simulink model "MZ0x2DH1921_EV_Personalise_design_witthmotor"  (R2023b)
settings: Solver=VariableStepAuto  StartTime=0.0  StopTime=100  RelTol=1e-3
libraries: spsDCVoltageSourceLib x3, spsDCMachineLib x2, spsControlledVoltageSourceLib x1, sps_lib x1
settings Model: Creator=HP5CD  LastModifiedBy=HP5CD

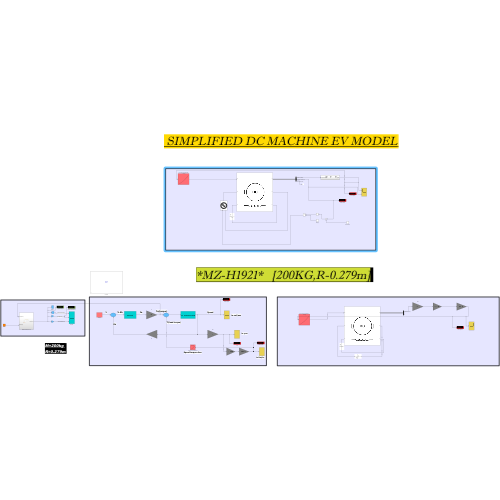
[thumbnail: Simulink's stored preview of the top-level diagram]
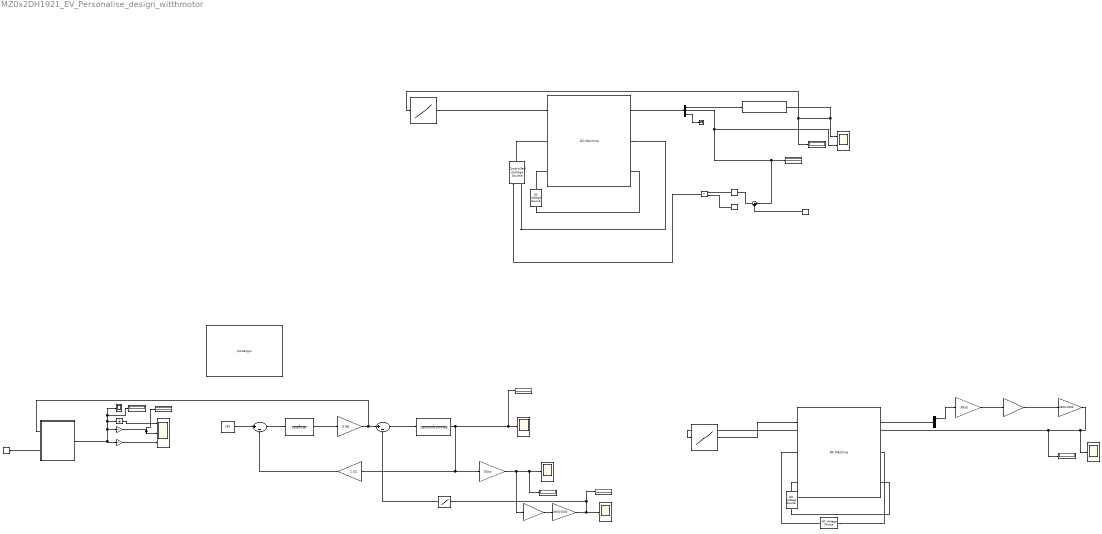
== system MZ0x2DH1921_EV_Personalise_design_witthmotor ==
  note: SIMPLIFIED DC MACHINE EV MODEL
  note: Speed torque-char
  note: in Km/hr
  note: in rpm
  note: in rad/sec
  note: Speed
  note: Tl(load torque)
  note: Te(torque)
  note: Ia
  note: V-Eb
  note: Eb
  note: V
  note: *MZ-H1921* [200KG,R-0.279m]
  note: Distance Covered(m)
  note: M=200kg
      | R=0.279m
  note: Speed(Km/hr)
  "                " : Gain  Gain=3600/1000
  "                Wheel RPM(no gear)" : Gain  Gain=60/(2.3*2*0.279)
  200KG Vehicle ,R=0.279 : Subsystem
  Bus Selector : BusSelector  OutputSignals=Speed wm (rad/s),Armature current ia (A),Field current if (A)
  Bus Selector1 : BusSelector  OutputSignals=Speed wm (rad/s),Armature current ia (A),Field current if (A)
  Controlled Voltage Source : spsControlledVoltageSourceLib/Controlled Voltage Source  Initialize=on  Source_Type=AC  Amplitude=0  Phase=0  Frequency=0  Measurements=None
  DC Machine : spsDCMachineLib/DC Machine  PresetModel=No  MechanicalLoad=Torque TL  FieldType=Wound  ShowDetailedParameters=on  MeasurementBus=off  RLa="[ 2.581  0.028]"  RLf="[ 281.3  3.156]"  Laf=0.9483  MachineConstant=Torque constant (N.m/A)  Ke=1.8  Kt=1.8  J=200*0.279*0.279  Bm=0.002953  Tf=0.5161  w0=1  Ifinit=0.853181656594383  TsPowergui=0  TsBlock=-1
  DC Machine1 : spsDCMachineLib/DC Machine  PresetModel=No  MechanicalLoad=Torque TL  FieldType=Wound  ShowDetailedParameters=on  MeasurementBus=off  RLa="[ 2.581  0.028]"  RLf="[ 281.3  3.156]"  Laf=0.9483  MachineConstant=Torque constant (N.m/A)  Ke=1.8  Kt=1.8  J=200*0.279*0.279  Bm=0.002953  Tf=0.5161  w0=1  Ifinit=0.853181656594383  TsPowergui=0  TsBlock=-1
  DC Voltage Source : spsDCVoltageSourceLib/DC Voltage Source  Amplitude=240  Measurements=None
  DC Voltage Source1 : spsDCVoltageSourceLib/DC Voltage Source  Amplitude=240  Measurements=None
  DC Voltage Source2 : spsDCVoltageSourceLib/DC Voltage Source  Amplitude=240  Measurements=None
  Gain : Gain  Gain=3600/1000
  Gain1 : Gain  Gain=(2*pi*0.279)/60
  Gain3 : Gain  Gain=3600/1000
  Gain4 : Gain  Gain=(2*pi*0.279)/60
  Integrator1 : Integrator
  Product : Product
  "Ref Current " : Constant  Value=20.5
  Relay : Relay  OnSwitchValue=1  OffSwitchValue=-1
  Scope{,1,3..4} (4 alike) : Scope
  Scope 1 : Scope
  Scope2 : Scope  NumInputPorts=3
  Scope5 : Scope  NumInputPorts=2
  Speed Display : Display
  Speed Display(KM/Hr) : Display
  Subsystem : Subsystem
  Sum : Sum  Inputs=|+-
  Sum1 : Sum  Inputs=|+-
  Sum2 : Sum  Inputs=|-+
  Terminator : Terminator
  Transfer Fcn : TransferFcn  Denominator=[0.028 2.581]
  Transfer Fcn1 : TransferFcn  Denominator=[(200*0.279*0.279) 0.003]
  Voltage : Constant  Value=110
  beta : Constant  Value=0
  kb : Gain  Gain=1.02
  kb1 : Gain  Gain=30/pi
  kb2 : Gain  Gain=30/pi
  km/hr speed{,1..3} (4 alike) : Display
  kt : Gain  Gain=0.98
  powergui : sps_lib/powergui  Priority=1  SimulationMode=Discrete  SampleTime=50e-6  frequency=60  Iterations=50  frequencyindice=0  Pbase=100e6  ErrMax=1e-4  UnitsV=kV  UnitsW=MW  buscounter=0  FunctionMessages=off  echomessages=off  EnableUseOfTLC=off  CurrentSourceSwitches=off  DisableSnubberDevices=off  DisableRonSwitches=off  DisableVfSwitches=off  DisplayEquations=off  AutomaticDiscreteSolvers=off  SolverType=Tustin/Backward Euler (TBE)  Interpol=off  ExternalGateDelay=off  methode=off  Ts=100  x0status=blocks  SPID=on  SwTol=0  HookPort=off  NonlinearTolerance=1e-4  nMaxIteration=100  ContinueOnMaxIteration=off  RestoreLinks=warning  ResistiveCurrentMeasurement=off  Frange=[0:2:500]  Ylog=off  Xlog=on  ShowGrid=off  save=off  variable=ZData  structure=0  ZoomFFT=off  StartTime=0.0  cycles=1  DisplayStyle=1  fundamental=60  FreqAxis=off  MaxFrequency=1000  frequencyindicesteady=1  RmsSteady=1  display=off
  rad/sec speed : Display
  rpm : Display
  torque speed characterstic : Lookup_n-D  NumberOfTableDimensions=1  BreakpointsForDimension1=[28.4, 40.16, 49.39, 56.8, 63.5, 69.56]  Table=[5, 10, 15, 20, 25, 30]  InternalRulePriority=Speed  RndMeth=Simplest
  torque speed characterstic1 : Lookup_n-D  NumberOfTableDimensions=1  BreakpointsForDimension1=[28.4, 40.16, 49.39, 56.8, 63.5, 69.56]  Table=[5, 10, 15, 20, 25, 30]  InternalRulePriority=Speed  RndMeth=Simplest
  torque speed characterstic2 : Lookup_n-D  NumberOfTableDimensions=1  BreakpointsForDimension1=[28.4, 40.16, 49.39, 56.8, 63.5, 69.56]  Table=[5, 10, 15, 20, 25, 30]  InternalRulePriority=Speed  RndMeth=Simplest
  voltage : Constant  Value=240
  wires:
  Integrator1/1 -> Scope2/1
  "                Wheel RPM(no gear)"/1 -> Scope2/3
  "                "/1 -> Speed Display(KM/Hr)/1, Scope2/2
  200KG Vehicle ,R=0.279/1(Speed(m/s)) -> Integrator1/1, Speed Display/1, Scope 1/1, "                "/1, "                Wheel RPM(no gear)"/1
  beta/1 -> 200KG Vehicle ,R=0.279/2(Beta(angle))
  Sum1/1 -> Transfer Fcn1/1
  Transfer Fcn1/1 -> kb/1, kb1/1, rad/sec speed/1, Scope/1
  Transfer Fcn/1 -> kt/1
  Sum/1 -> Transfer Fcn/1
  voltage/1 -> Sum/1
  kb/1 -> Sum/2
  kb1/1 -> Gain1/1, rpm/1, Scope1/1
  Gain1/1 -> Gain/1
  Gain/1 -> km/hr speed/1, torque speed characterstic/1, Scope3/1
  torque speed characterstic/1 -> Sum1/2
  kt/1 -> 200KG Vehicle ,R=0.279/1(Torque(N-m)), Sum1/1
  DC Machine/1 -> Bus Selector/1
  Gain4/1 -> Gain3/1
  Bus Selector/1 -> kb2/1  "<Speed wm (rad/s)>"
  torque speed characterstic1/1 -> DC Machine/1
  kb2/1 -> Gain4/1
  Gain3/1 -> Scope4/1, km/hr speed1/1, torque speed characterstic1/1
  torque speed characterstic2/1 -> DC Machine1/1
  DC Machine1/1 -> Bus Selector1/1
  Subsystem/1(KM/HR) -> Scope5/1, km/hr speed2/1, torque speed characterstic2/1
  Bus Selector1/1 -> Subsystem/1(<Speed wm (rad/s)>)  "<Speed wm (rad/s)>"
  Bus Selector1/2 -> Scope5/2, Sum2/1, km/hr speed3/1  "<Armature current ia (A)>"
  Voltage/1 -> Product/2
  Relay/1 -> Product/1
  "Ref Current "/1 -> Sum2/2
  Sum2/1 -> Relay/1
  Product/1 -> Controlled Voltage Source/1
  Bus Selector1/3 -> Terminator/1  "<Field current if (A)>"
  connections:
  DC Voltage Source/RConn1 -- DC Machine/LConn2
  DC Voltage Source/LConn1 -- DC Machine/RConn2
  DC Voltage Source1/RConn1 -- DC Machine/LConn1
  DC Voltage Source1/LConn1 -- DC Machine/RConn1
  DC Voltage Source2/RConn1 -- DC Machine1/LConn2
  DC Voltage Source2/LConn1 -- DC Machine1/RConn2
  Controlled Voltage Source/RConn1 -- DC Machine1/LConn1
  DC Machine1/RConn1 -- Controlled Voltage Source/LConn1

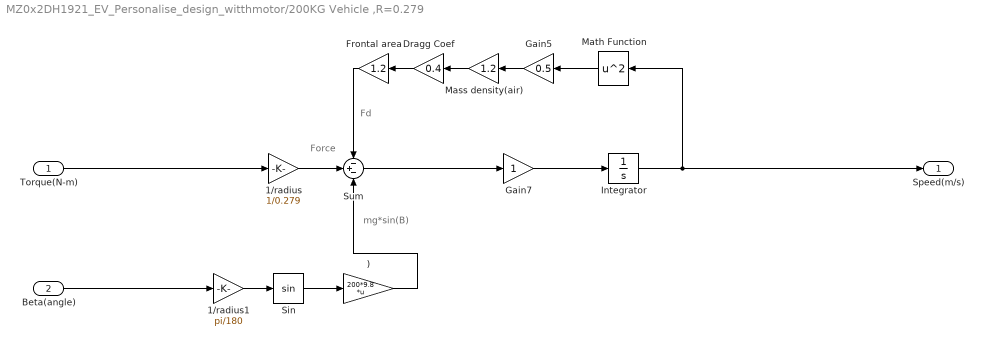
== system MZ0x2DH1921_EV_Personalise_design_witthmotor/200KG Vehicle ,R=0.279 ==
  note: Force
  note: mg*sin(B)
  note: Fd
  Torque(N-m) : Inport
  Beta(angle) : Inport  Port=2
  ) : Gain  Gain=200*9.8  Multiplication=Matrix(K*u)
  1/radius : Gain  Gain=1/0.279
  1/radius1 : Gain  Gain=pi/180
  Dragg Coef : Gain  Gain=0.4
  Frontal area : Gain  Gain=1.2
  Gain5 : Gain  Gain=0.5
  Gain7 : Gain
  Integrator : Integrator
  Mass density(air) : Gain  Gain=1.2
  Math Function : Math  Operator=square
  Sin : Trigonometry
  Sum : Sum  Inputs=-+-
  Speed(m/s) : Outport
  wires:
  1/radius/1 -> Sum/2
  Integrator/1 -> Speed(m/s)/1, Math Function/1
  Dragg Coef/1 -> Frontal area/1
  )/1 -> Sum/3
  Mass density(air)/1 -> Dragg Coef/1
  Math Function/1 -> Gain5/1
  Sum/1 -> Gain7/1
  Sin/1 -> )/1
  Gain7/1 -> Integrator/1
  Gain5/1 -> Mass density(air)/1
  1/radius1/1 -> Sin/1
  Frontal area/1 -> Sum/1
  Torque(N-m)/1 -> 1/radius/1
  Beta(angle)/1 -> 1/radius1/1

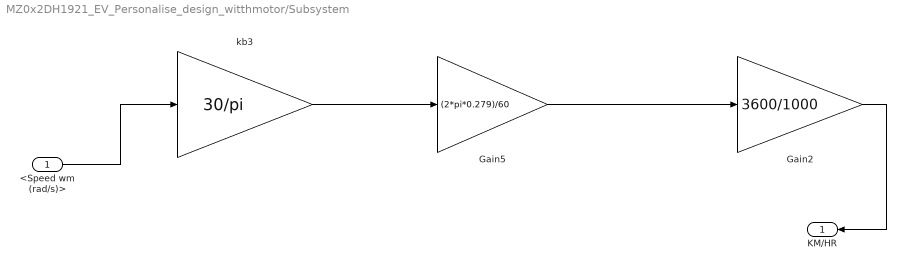
== system MZ0x2DH1921_EV_Personalise_design_witthmotor/Subsystem ==
  <Speed wm (rad/s)> : Inport
  Gain2 : Gain  Gain=3600/1000
  Gain5 : Gain  Gain=(2*pi*0.279)/60
  kb3 : Gain  Gain=30/pi
  KM/HR : Outport
  wires:
  <Speed wm (rad/s)>/1 -> kb3/1
  kb3/1 -> Gain5/1
  Gain5/1 -> Gain2/1
  Gain2/1 -> KM/HR/1
